simulink model "v00_0A_0D"  (R2022b)
settings: Solver=FixedStepDiscrete  StartTime=0.0  StopTime=8000  FixedStep=SampleTime  MaxStep=Contactors_StepTime_msec  RelTol=1e-3  EnableMultiTasking=on
undefined symbols (not defined in the file): A_to_mA, BalancingTempGroup, canChannel, CapacityFactor, CC_Inputs, CellSOC, ChargeState, ContactorsFlags, DiscIntNeverNeededParam, gEN_Contactors_StepTime_msec, Ion, isDynamicCurrentEn, Lithium, maxAllowedImbalance, nCells_parallel, nCells_series, nCellTempGrps, PermanentFailRecoveryTrigger, ProtectionFlags, RBal_ohm, SampleTime, sigbuilder_block, StLineEq_varA, StLineEq_varB, TempSelectForDCL, Thresholds, V_to_mV
libraries: simulink x32, spsIdealSwitchLib x21, spsBatteryLib x20, spsSeriesRLCBranchLib x20, spsVoltageMeasurementLib x20, canmsglib x4, canlib x3, dspstat3 x2, spspowerguiLib x2, spsControlledCurrentSourceLib x1, spsCurrentMeasurementLib x1
(part 7 of 7)

== stateflow chart v00_0A_0D/HighLevelStatemachine/HighLevelStatemachine ==
  state HighLevelStatemachine [parallel]
    settings: executionOrder=1
    state Normal_Mode [group]
      state Idle
        entry: HighLevelState = HighLevelMode.Idle;
      state Discharging
        entry: HighLevelState = HighLevelMode.Discharging;
      state FastCharging
        entry: HighLevelState = HighLevelMode.ChargingFast;
      state SlowCharging
        entry: HighLevelState = HighLevelMode.ChargingSlow;
      state Regeneration
        entry: HighLevelState = HighLevelMode.Regeneration;
      (default) -> HighLevelStatemachine.Normal_Mode.Idle
      HighLevelStatemachine.Normal_Mode.Idle -> Discharging [order 1] : [duration(DataPipeline.isChargeEn ==0, msec)>Thresholds.NormalModeTimeout_msec]
      Discharging -> HighLevelStatemachine.Normal_Mode.Idle [order 2] : [duration(DataPipeline.Current_mA < Thresholds.ChargeDetectionThreshold_mA, msec) > Thresholds.NormalModeTimeout_msec]
      FastCharging -> Discharging [order 3] : [duration(DataPipeline.isChargeEn ==0, msec)>Thresholds.NormalModeTimeout_msec]
      FastCharging -> HighLevelStatemachine.Normal_Mode.Idle [order 2] : [duration(DataPipeline.Current_mA < Thresholds.ChargeDetectionThreshold_mA, msec) > Thresholds.NormalModeTimeout_msec]
      Discharging -> SlowCharging [order 1] : [duration(DataPipeline.isChargeEn ==1, msec)>Thresholds.NormalModeTimeout_msec]
      SlowCharging -> Discharging [order 4] : [duration(DataPipeline.isChargeEn ==0, msec)>Thresholds.NormalModeTimeout_msec]
      Discharging -> Regeneration [order 3] : [duration((DataPipeline.VCU.isChargerConnected == 0 && DataPipeline.isChargeEn ==1), msec)>Thresholds.NormalModeTimeout_msec]
      Regeneration -> Discharging [order 1] : [duration(DataPipeline.isChargeEn == 0, msec)> Thresholds.NormalModeTimeout_msec]
      HighLevelStatemachine.Normal_Mode.Idle -> SlowCharging [order 2] : [duration(DataPipeline.isChargeEn ==1, msec)>Thresholds.NormalModeTimeout_msec]
      SlowCharging -> HighLevelStatemachine.Normal_Mode.Idle [order 2] : [duration(DataPipeline.Current_mA < Thresholds.ChargeDetectionThreshold_mA, msec) > Thresholds.NormalModeTimeout_msec]
      SlowCharging -> FastCharging [order 1] : [duration(DataPipeline.VCU.FastCharge == 1, msec)>Thresholds.NormalModeTimeout_msec ]
      FastCharging -> SlowCharging [order 1] : [duration(DataPipeline.VCU.SlowCharge == 1, msec)>Thresholds.NormalModeTimeout_msec ]
    state PowerSaver_Mode [group]
      state LowPowerMode
        entry: HighLevelState = HighLevelMode.LowPowerMode;
      state DeepSleepMode
        entry: HighLevelState = HighLevelMode.DeepSleepMode;
      LowPowerMode -> DeepSleepMode : [duration(HighLevelState == HighLevelMode.LowPowerMode, msec) > Thresholds.PowerSaverModeTimeout_msec]
    state Fault_Mode
      state PermanentFailure
        HighLevelState = HighLevelMode.PermanentFailFault;
      state Protection
        HighLevelState = HighLevelMode.ProtectionFault;
      state LimpHome
        HighLevelState = HighLevelMode.LimpHomeFault;
      LimpHome -> PermanentFailure [order 1] : [duration(DataPipeline.VCU.VCUPermanentFail ==1, msec)> Thresholds.FaultsModeTimeout_msec]
      Protection -> LimpHome [order 1] : [duration(DataPipeline.VCU.TransmissionFail ==1 , msec)> Thresholds.FaultsModeTimeout_msec]
    state Service_Mode [group]
      state ServiceMode
        entry: HighLevelState = HighLevelMode.ServiceMode;
    HighLevelStatemachine.Normal_Mode.Idle -> ServiceMode [order 4] : [duration(DataPipeline.VCU.ServiceMode==1,msec)>Thresholds.ServiceModeTimeout_msec]
    Discharging -> Protection [order 4] : [duration(ProtectionOutput.ErrorDetect ==1,msec)>Thresholds.FaultsModeTimeout_msec]
    HighLevelStatemachine.Normal_Mode.Idle -> LowPowerMode [order 3] : [duration(HighLevelState == HighLevelMode.Idle, msec) > Thresholds.PowerSaverModeTimeout_msec]
    FastCharging -> Protection [order 4] : [duration(ProtectionOutput.ErrorDetect ==1,msec)>Thresholds.FaultsModeTimeout_msec]
    SlowCharging -> Protection [order 3] : [duration(ProtectionOutput.ErrorDetect ==1,msec)>Thresholds.FaultsModeTimeout_msec]
    Regeneration -> Protection [order 2] : [duration(ProtectionOutput.ErrorDetect ==1,msec)>Thresholds.FaultsModeTimeout_msec]
    PermanentFailure -> ServiceMode : [duration(DataPipeline.VCU.ServiceMode==1,msec)>Thresholds.ServiceModeTimeout_msec]
    DeepSleepMode -> ServiceMode : [duration(DataPipeline.VCU.ServiceMode==1,msec)>Thresholds.ServiceModeTimeout_msec]
    Protection -> ServiceMode [order 2] : [duration(DataPipeline.VCU.ServiceMode==1,msec)>Thresholds.ServiceModeTimeout_msec]
    LimpHome -> ServiceMode [order 2] : [duration(DataPipeline.VCU.ServiceMode==1,msec)>Thresholds.ServiceModeTimeout_msec]
  state BMS_State [parallel]
    settings: executionOrder=2
    state Idle
    state Ready
      en:
      BMS_State = BMSState.MARVEL_READY;
    state Activating
      en:
      BMS_State = BMSState.MARVEL_ACTIVATING;
    state Error
      en:
      BMS_State = BMSState.MARVEL_ERROR;
    state Active
      en:
      BMS_State = BMSState.MARVEL_ACTIVE;
    (default) -> BMS_State.Idle
    BMS_State.Idle -> Activating [order 2] : [ContactorCommand==1]
    BMS_State.Idle -> Ready [order 1] : [ContactorCommand==0]
    Ready -> Activating [order 1] : [ContactorsState > 0 && ContactorCommand==1]
    Activating -> Ready [order 3] : [ContactorCommand==0&& ContactorsState==0]
    Activating -> Error [order 2] : [duration(ContactorCommand==1&& (ContactorsState==0 || ContactorsState==8),msec)>Thresholds.BMS_ActivatingToError_Timeout_msec]
    Error -> Ready [order 1] : [ProtectionOutput.ErrorDetect == ProtectionFlags.NoError && ContactorsState == 0 && ContactorCommand==0]
    Ready -> Error [order 2] : [ProtectionOutput.ErrorDetect == ProtectionFlags.Error || ContactorsState >6]
    Active -> Ready [order 2] : [ContactorCommand==0&&ContactorsState~=5]
    Error -> Activating [order 2] : [duration((ContactorCommand==1&&ContactorsState>0&&ContactorsState<=6),msec)>Thresholds.BMS_ErrorToActivating_Timeout_msec]
    Activating -> Active [order 1] : [ContactorsState == 5]
    Active -> Activating [order 3] : [ContactorsState<6 && ContactorCommand==1 && ContactorsState~=5]
    Active -> Error [order 1] : [ContactorCommand==1&&(ContactorsState==0||ContactorsState==8)]
  data: Thresholds input; ContactorCommand input; ContactorsState input; ProtectionOutput input; HighLevelState output Enum: HighLevelMode =HighLevelMode.Idle; DataPipeline input; BMS_State output

== matlab function v00_0A_0D/DataPipeline/AverageFunction ==
  data: u1 input; u2 input; Average output; n input
function Average  = fcn(u1,u2,n)
A = [u1,u2];
Average = mean(A(1:n));
end

== matlab function v00_0A_0D/DataPipeline/MaximumFunction ==
  data: n input; u1 input; u2 input; Max output
function Max  = fcn(n,u1,u2)
A = [u1,u2];
Max = max(A(1:n));
end

== matlab function v00_0A_0D/DataPipeline/DynamicCurrentLimits_perParallelCell ==
  data: DCL_ChargingCurrent_A output; DCL_DisChargingCurrent_A output; DCL_arcReactor_A output; SOC input; Temperature_C input
 function [DCL_ChargingCurrent_A, DCL_DisChargingCurrent_A, DCL_arcReactor_A]= fcn(SOC,Temperature_C)
% DCL_ChargingCurrent_A = (SOC*Temperature_C/20);
% DCL_DisChargingCurrent_A = (SOC*Temperature_C/20);
DCL_ChargingCurrent_A = 120;
DCL_DisChargingCurrent_A = (SOC*Temperature_C/20);
DCL_arcReactor_A = (12);
end

== matlab function v00_0A_0D/DataPipeline/MinimumFunction ==
  data: n input; u1 input; u2 input; Min output
function Min  = fcn(n,u1,u2)
A = [u1,u2];
Min = min(A(1:n));
end

== stateflow chart v00_0A_0D/SOCEstimation/CoulombCounter/Chart1 ==
  state IntegratedCurrent
    during:
    IntegratedCurrent = single(single(LoopTimer_SOC_msec)*single(Current_mA))+IntegratedCurrent;
  state IntegratorReset
    during:
    IntegratedCurrent = 0;
  (default) -> IntegratedCurrent
  IntegratedCurrent -> IntegratorReset : [CC_State ==1]
  IntegratorReset -> IntegratedCurrent : [CC_State ==0 || CC_State ==2]
  data: LoopTimer_SOC_msec input; Current_mA input; IntegratedCurrent output =single(0); CC_State input

== stateflow chart v00_0A_0D/SOCEstimation/SOC_Calibration/SOC_Calibration ==
  state Vehicle_at_Rest
    entry:  CC_State = CCState.Vehicle_at_Rest; % CC_State == 2;
    Initial_Capacity_mAh = int32(Initial_Guess_mAh);
    TransitionCapacity_mAh = Initial_Capacity_mAh;
  state CoulombCounting
    entry:
    CC_State = CCState.CoulombCounting; % CC_State == 0;
    Initial_Capacity_mAh = int32(Capacity_mAh);
    during:
    DeltaCapacity_mAh = int32(abs(Initial_Capacity_mAh - TransitionCapacity_mAh));
  state PseudoLatchHandler
    entry:
    pseudoLatchSuccess = false;
  note: It has to be ensured that at a condition at the following conditions:
      | MaxVoltageLimit_mV
      | MaxCurrentLimit_mA
      | MinCurrentLimit_mA
      | There must be sufficient capacity available in the pack to enable the
      | CapacityDeltaCheck_mAh condition.
  note: [duration(DataPipeline.VoltageSenseBus.mV_min>=(single(CC_Inputs.MaxVoltageLimit_mV) - single(CC_Inputs.MaxAllowedImb_mV)),msec)>CC_Inputs.DebouncingTimeout_msec && DataPipeline.VCU.isChargerConnected == 1 && CellBalancingOutput.MaxImbalance_mV<CC_Inputs.MaxAllowedImb_mV && (duration((abs(Current_mA)<CC_Inputs.MaxCurrentLimit_mA && abs(Current_mA)>CC_Inputs.MinCurrentLimit_mA),msec)>CC_Inputs.DebouncingTimeout_msec)]
  state Recalibrate_Charging
    entry:
    CC_State = CCState.Recalibrate; % CC_State == 1;
    Initial_Capacity_mAh = int32(MaxUsableCapacity_mAh);
    TransitionCapacity_mAh = Initial_Capacity_mAh;
  note: should make pseudoLatchSuccess false after calibration
  (default) -> Vehicle_at_Rest
  CoulombCounting -> PseudoLatchHandler [order 2] : [pseudoLatchSuccess == true]
  Vehicle_at_Rest -> CoulombCounting : [after(CC_Inputs.CCTimeout_msec, msec)]
  Recalibrate_Charging -> CoulombCounting : [after(CC_Inputs.CCTimeout_msec, msec)]
  CoulombCounting -> Recalibrate_Charging [order 1] : [duration(((DataPipeline.VoltageSenseBus.mV_min>=minVoltageForLatch) && (abs(Current_mA)<MaxCurrentLimit_mA && abs(Current_mA)>MinCurrentLimit_mA)),msec)>DebouncingTimeout_msec && DataPipeline.VCU.isChargerConnected == 1 && CellBalancingOutput.MaxImbalance_mV<MaxAllowedImb_mV]
  PseudoLatchHandler -> Recalibrate_Charging
  data: MinCurrentLimit_mA input; MaxUsableCapacity_mAh input; Initial_Guess_mAh input; Current_mA input; CC_Inputs input; DataPipeline input; CellBalancingOutput input; CC_State output Enum: CCState; pseudoLatchSuccess output; Capacity_mAh input; Initial_Capacity_mAh output int32; DeltaCapacity_mAh local; TransitionCapacity_mAh local; minVoltageForLatch input; MaxAllowedImb_mV input; MaxCurrentLimit_mA input; DebouncingTimeout_msec input; pseudoLatchSuccess input

== matlab function v00_0A_0D/DataPipeline/I2t_perParallelCell ==
  data: SOC input; i2t_Charge_A2sec output; Temperature_C input; i2t_Discharge_A2sec output
function [i2t_Charge_A2sec, i2t_Discharge_A2sec]= fcn(SOC,Temperature_C)
    i2t_Charge_A2sec = (SOC*Temperature_C*128);
    i2t_Discharge_A2sec = (SOC*Temperature_C*12);
    % i2t_Charge_mA2msec = SOC*Temperature_C*12;
    % i2t_Discharge_mA2msec = SOC*Temperature_C*12;
end

== matlab function v00_0A_0D/SOCEstimation/SOC_ReadFromFlash ==
  data: CapacityRemains_mAh output
function CapacityRemains_mAh = fcn
w = 165; % random value for trial
CapacityRemains_mAh = int32(w * 1000);
end

== matlab function v00_0A_0D/SOCEstimation/SOC_WriteToFlash ==
  data: A output; SOH_pct input; TotalCapacityExchange_mAh input; MaxUsableCapacity_mAh input; SOC_cpct input; TotalDischarge_mAh input; TotalCapacityRemains_mAh input; XYZ output; SOC output
  function [A,XYZ,SOC] = fcn(SOH_pct,TotalCapacityExchange_mAh, MaxUsableCapacity_mAh,SOC_cpct, TotalDischarge_mAh, TotalCapacityRemains_mAh)
A = single(SOH_pct)*single(TotalDischarge_mAh);
B = single(TotalCapacityExchange_mAh)/single(MaxUsableCapacity_mAh);
C = single(SOC_cpct)-single(TotalCapacityRemains_mAh);
XYZ = A+B+C;
SOC = SOC_cpct;
end

== stateflow chart v00_0A_0D/SOCEstimation/SOH_Calculation/Chart ==
  state IntegratedCurrent
    during:
    IntegratedCurrent = single(single(LoopTimer_SOC_msec)*single(Current_mA))+IntegratedCurrent;
  (default) -> IntegratedCurrent
  data: LoopTimer_SOC_msec input; Current_mA input; IntegratedCurrent output =single(0)

== matlab function v00_0A_0D/SOCEstimation/SOH_Calculation/UsableCapacity_mAh ==
  data: CycleCount input; SOH_Vs_Capacity_Gain input; SOH_Vs_Capacity_Offset input; MaxUsableCapacity_mAh output; InstalledCapacity_mAh input
function MaxUsableCapacity_mAh = fcn(CycleCount, SOH_Vs_Capacity_Gain, SOH_Vs_Capacity_Offset, InstalledCapacity_mAh)
    MaxUsableCapacity_mAh = int32(single(InstalledCapacity_mAh) - (single(SOH_Vs_Capacity_Gain) * (single(CycleCount) + single(SOH_Vs_Capacity_Offset))));
end

== stateflow chart v00_0A_0D/SOCEstimation/SOH_Calibration/SOH_Calibration ==
  state TestBench_Entry
    entry: CycleCompleted = 0;
  state Full_Charge
    entry: CycleCompleted = CycleCompleted + 0.5;
  state Int3
  state Int4
  state Full_Discharge
    entry: CycleCompleted = CycleCompleted + 0.5;
  state Int1
  state Int2
  (default) -> TestBench_Entry
  Int3 -> TestBench_Entry [order 2] : [duration(DataPipeline.isChargeEn == 0,msec)>=CC_Inputs.SOHCalibrationTimeout_msec]{CalcEnable = 0}
  Int3 -> Full_Charge [order 1] : [duration(ProtectionOutput.OV == ProtectionFlags.Error,msec)>=CC_Inputs.SOHCalibrationTimeout_msec]{CalcEnable = 1}
  TestBench_Entry -> Int3 [order 2] : [duration(DataPipeline.isChargeEn == 1,msec)>=CC_Inputs.SOHCalibrationTimeout_msec]{CalcEnable = 1}
  Full_Charge -> TestBench_Entry [order 2] : [duration(DataPipeline.isChargeEn == 0 && ProtectionOutput.OV ~= ProtectionFlags.Error,msec)>=CC_Inputs.SOHCalibrationTimeout_msec]{CalcEnable = 0}
  TestBench_Entry -> Int4 [order 1] : [duration(DataPipeline.isChargeEn == 0,msec)>=CC_Inputs.SOHCalibrationTimeout_msec]{CalcEnable = 1}
  Int4 -> TestBench_Entry [order 2] : [duration(DataPipeline.isChargeEn == 1,msec)>=CC_Inputs.SOHCalibrationTimeout_msec]{CalcEnable = 0}
  Full_Discharge -> TestBench_Entry [order 2] : [duration(DataPipeline.isChargeEn == 1 && ProtectionOutput.UV ~= ProtectionFlags.Error,msec)>=CC_Inputs.SOHCalibrationTimeout_msec]{CalcEnable = 0}
  Int2 -> TestBench_Entry [order 1] : [duration(DataPipeline.isChargeEn == 1,msec)>=CC_Inputs.SOHCalibrationTimeout_msec]{CalcEnable = 0}
  Int1 -> TestBench_Entry [order 2] : [duration(DataPipeline.isChargeEn == 0,msec)>=CC_Inputs.SOHCalibrationTimeout_msec]{CalcEnable = 0}
  Int1 -> Full_Charge [order 1] : [duration(DataPipeline.isChargeEn == 0 && ProtectionOutput.OV == ProtectionFlags.Error, msec) >= CC_Inputs.SOHCalibrationTimeout_msec]{CalcEnable = 1}
  Full_Charge -> Int2 [order 1] : [duration(DataPipeline.isChargeEn == 0,msec)>=CC_Inputs.SOHCalibrationTimeout_msec]{CalcEnable = 1}
  Int4 -> Full_Discharge [order 1] : [duration(ProtectionOutput.UV == ProtectionFlags.Error,msec)>=CC_Inputs.SOHCalibrationTimeout_msec]{CalcEnable = 1}
  Full_Discharge -> Int1 [order 1] : [duration(DataPipeline.isChargeEn == 1,msec)>=CC_Inputs.SOHCalibrationTimeout_msec]{CalcEnable = 1}
  Int2 -> Full_Discharge [order 2] : [duration(DataPipeline.isChargeEn == 0 && ProtectionOutput.UV == ProtectionFlags.Error,msec)>=CC_Inputs.SOHCalibrationTimeout_msec]{CalcEnable = 1}
  data: ProtectionOutput input; CC_Inputs input; DataPipeline input; CalcEnable output; CycleCompleted output

== stateflow chart v00_0A_0D/SOCEstimation/SOH_Calibration/Subsystem/Chart ==
  state IntegratedCurrent
    during:
    IntegratedCurrent = single(single(LoopTimer_SOC_msec)*single(Current_mA))+IntegratedCurrent;
  state Reset_IntegratedCurrent
    entry:
    Final_IntegratedCurrent = IntegratedCurrent;
  (default) -> IntegratedCurrent
  IntegratedCurrent -> Reset_IntegratedCurrent : [duration(CycleCompleted == 1,msec)>=CC_Inputs.SOHCalibrationTimeout_msec]
  Reset_IntegratedCurrent -> IntegratedCurrent : [duration(CycleCompleted == 0, msec)>=CC_Inputs.SOHCalibrationTimeout_msec]{IntegratedCurrent = 0}
  data: LoopTimer_SOC_msec input; Current_mA input; CycleCompleted input; CC_Inputs input; Final_IntegratedCurrent output; IntegratedCurrent local =single(0)

== matlab function v00_0A_0D/SOCEstimation/SOH_Calibration/Subsystem/UsableCapacity_mAh ==
  data: CycleCount input; MaxUsableCapacity_mAh output; InstalledCapacity_mAh input; SOH_Vs_Capacity_Gain input; SOH_Vs_Capacity_Offset input
function MaxUsableCapacity_mAh = fcn(CycleCount, InstalledCapacity_mAh, SOH_Vs_Capacity_Gain, SOH_Vs_Capacity_Offset)
    MaxUsableCapacity_mAh = int32(single(InstalledCapacity_mAh) - (single(SOH_Vs_Capacity_Gain) * (single(CycleCount) + single(SOH_Vs_Capacity_Offset))));
end

== matlab function v00_0A_0D/SOCEstimation/Voltage_Vs_Capacity ==
  data: Voltage_mV input; Capacity_mAh output
function Capacity_mAh = fcn(Voltage_mV)

Capacity_mAh = uint32(Voltage_mV*50);

== stateflow chart v00_0A_0D/SOCEstimation/Chart ==
  state Lobby
    entry: Final_InstalledCapacity_mAh = CC_Inputs.InstalledCapacity_mAh;
  state FirstCycleCompleted
    entry: Final_InstalledCapacity_mAh = Tested_InstalledCapacity_mAh;
  (default) -> Lobby
  Lobby -> FirstCycleCompleted : [duration(CC_Inputs.SOHCalibrationOn == true && CycleCompleted == 1,msec)>CC_Inputs.DebouncingTimeout_msec]
  FirstCycleCompleted -> Lobby : [CC_Inputs.SOHCalibrationOn == false]
  data: CycleCompleted input; Final_InstalledCapacity_mAh output int32; Tested_InstalledCapacity_mAh input; CC_Inputs input

== stateflow chart v00_0A_0D/CellBalancing/InputProcessing/Chart1 ==
  state PCBTemp_Safe
    entry: PCBTemp = true;
  state PCBTemp_Danger
    entry: PCBTemp = false;
  (default) -> PCBTemp_Safe
  PCBTemp_Safe -> PCBTemp_Danger : [DataPipeline.TemperatureSenseBus(2).T_max >= Thresholds.Temperature(2).Protections_OTC_Error_C || DataPipeline.TemperatureSenseBus(2).T_max >= Thresholds.Temperature(2).Protections_OTD_Error_C]
  PCBTemp_Danger -> PCBTemp_Safe : [DataPipeline.TemperatureSenseBus(2).T_max < Thresholds.Temperature(2).Protections_OTC_Error_C || DataPipeline.TemperatureSenseBus(2).T_max < Thresholds.Temperature(2).Protections_OTD_Error_C]
  data: Thresholds input; DataPipeline input; PCBTemp output

== stateflow chart v00_0A_0D/SOCEstimation/CoulombCounter/Chart ==
  state Lobby
    entry:
    during: TotalCapacityRemains_mAh = Initial_Capacity_mAh + IntegratedCurrent;
  state Zero_Charged
    during: TotalCapacityRemains_mAh = 0;
  state PseudoLatchHandler
    during: TotalCapacityRemains_mAh = Initial_Capacity_mAh + IntegratedCurrent;
  state Fully_Charged
    entry: TotalCapacityRemains_mAh = MaxUsableCapacity_mAh;
    during: TotalCapacityRemains_mAh = Initial_Capacity_mAh + IntegratedCurrent;
  (default) -> Lobby
  Lobby -> Zero_Charged [order 2] : [TotalCapacityRemains_mAh <= 0]
  Lobby -> PseudoLatchHandler [order 3] : [duration((pseudoLatchFlag == true && isChargeEn == 1),msec) > debounceTimeout]
  Zero_Charged -> Lobby : [isChargeEn==1]
  PseudoLatchHandler -> Lobby [order 2] : [duration(pseudoLatchFlag == 0,msec) > debounceTimeout]
  Lobby -> Fully_Charged [order 1] : [Initial_Capacity_mAh == MaxUsableCapacity_mAh && CC_State == 1 && pseudoLatchFlag == false]
  Fully_Charged -> Lobby : [CC_State == 0]
  PseudoLatchHandler -> Fully_Charged [order 1] : [duration(TotalCapacityRemains_mAh >= MaxUsableCapacity_mAh,msec) > debounceTimeout]{pseudoLatchSuccess = true}
  data: isChargeEn input; Initial_Capacity_mAh input; CC_State input; debounceTimeout input; IntegratedCurrent input; TotalCapacityRemains_mAh output =int32(2); MaxUsableCapacity_mAh input; pseudoLatchFlag input; pseudoLatchSuccess output

== stateflow chart v00_0A_0D/HearbeatMonitoring_Configuration/Chart ==
  state Hardware_NoError
    entry: HardwareError = ProtectionFlags.NoError;
  state Hardware_YesError
    entry: HardwareError = ProtectionFlags.Error;
  (default) -> Hardware_NoError
  Hardware_NoError -> Hardware_YesError : [duration(Status==0,msec)>=Thresholds.HardwareError_Timeout_msec]
  data: Status input; Thresholds input; HardwareError output

== stateflow chart v00_0A_0D/HeartbeatMonitoring_Initial/Chart ==
  state HeartbeatCheck_Normal
    entry:
    CAN_Transmission = ProtectionFlags.NoError;
  state HeartbeatCheck_Fail
    entry:
    CAN_Transmission = ProtectionFlags.PermanentFail;
  (default) -> HeartbeatCheck_Normal
  HeartbeatCheck_Normal -> HeartbeatCheck_Fail : [ClockTime > (HeartbeatCounter + 5)]
  data: HeartbeatCounter input; ClockTime input; CAN_Transmission output =ProtectionFlags.NoError

== stateflow chart v00_0A_0D/Protection/Chart ==
  state Integrator_On
    entry:
    m = 1;
    Trigger = 0;
  state Integrator_Reset
    entry:
    m = 0;
    Trigger = 1;
  (default) -> Integrator_On
  Integrator_On -> Integrator_Reset : [duration(m == 1,msec) == AverageTime_msec]
  Integrator_Reset -> Integrator_On : after(10,msec)
  data: Trigger output; m local =uint8(0); AverageTime_msec input

== stateflow chart v00_0A_0D/ChargingAlgorithm/IRCalc ==
  state IRLobby
    en:
    firstVolt = int32(0);
    secondVolt = int32(0);
    thirdVolt = int32(0);
    firstRequestedCurrent = int32(10);
    secondRequestedCurrent= int32(0);
    thirdRequestedCurrent= int32(0);
    internalResistancePulseCurrent = ChargingRequestedCurrent;
  state IRCalculation
    state ResetIRCycleCount
      du:
      if IRComplete == true
      EraseRecordedCycleCount = 1;
      end
    state IRCalcBegin
      du:
      firstRequestedCurrent = DataPipeline.Current_mA;
      firstVolt = DataPipeline.TerminalVoltage_mV;
      internalResistancePulseCurrent = ChargingRequestedCurrent;
    state UpSense
      du:
      thirdVolt = DataPipeline.TerminalVoltage_mV;
      thirdRequestedCurrent = DataPipeline.Current_mA;
    state DropPulse
      du:
      internalResistancePulseCurrent = 0;
    state DropSense
      du:
      secondVolt = DataPipeline.TerminalVoltage_mV;
      secondRequestedCurrent = DataPipeline.Current_mA;
      internalResistancePulseCurrent = ChargingRequestedCurrent;
    (default) -> IRCalcBegin
    UpSense -> ResetIRCycleCount : [after(Thresholds.IRTransition_msec,msec)]
    IRCalcBegin -> DropPulse : [after(Thresholds.IRTransition_msec,msec)]
    DropSense -> UpSense : [after(Thresholds.IRTransition_msec,msec)]
    DropPulse -> DropSense : [after(Thresholds.IRPulseDropTime_sec,sec)]
  state Entry
  (default) -> IRLobby
  IRLobby -> Entry
  Entry -> IRCalculation : [duration((DataPipeline.VCU.isChargerConnected==true &&...
      | (DataPipeline.VCU.SlowCharge==true ||....
      |  DataPipeline.VCU.FastCharge==true) && IRComplete == false),msec) >= Thresholds.IRTransition_msec]
  IRCalculation -> Entry : [duration((DataPipeline.VCU.isChargerConnected==false ||...
      | (DataPipeline.VCU.SlowCharge==false ||....
      |  DataPipeline.VCU.FastCharge==false)&& IRComplete == false),msec) >= Thresholds.IRTransition_msec]
  data: DataPipeline input; IRComplete input; Thresholds input; internalResistancePulseCurrent output; secondRequestedCurrent output; firstRequestedCurrent output; secondVolt output; firstVolt output; thirdVolt output; thirdRequestedCurrent output; ChargingRequestedCurrent input; EraseRecordedCycleCount output

== stateflow chart v00_0A_0D/ChargingAlgorithm/ChargingAlgorithmstep2 ==
  state chargingLobby
    en:
    Constant_K = double(0);
    trickleChargingEnabled = false;
  state TrickleCharging
    state TrickleChargeDisabled
      en:
      du:
      trickleChargingEnabled = false;
    state TrickleChargeEnabled
      en:
      du:
      trickleChargingEnabled = true;
    (default) -> TrickleChargeDisabled
    TrickleChargeDisabled -> TrickleChargeEnabled [order 1] : [DataPipeline.VoltageSenseBus.mV_min <= Thresholds.trickleChargingLimit]
    TrickleChargeEnabled -> TrickleChargeDisabled : [[DataPipeline.VoltageSenseBus.mV_min > Thresholds.trickleChargingLimit]]
  state NormalCharging
    du:
    state FastCharging
      en:
      du:
      state CC
        en:
        du:
        Constant_K = Thresholds.FastCharge_CC_K;
      state CV
        en:
        du:
        Constant_K = Thresholds.FastCharge_CV_K;
        cvModeActivated = true;
      (default) -> NormalCharging.FastCharging.CC
      NormalCharging.FastCharging.CC -> NormalCharging.FastCharging.CV : [DataPipeline.VoltageSenseBus.mV_max >= Thresholds.transitionVoltageCV]
    state SlowCharging
      en:
      du:
      state CC
        en:
        du:
        Constant_K = Thresholds.SlowCharge_CC_K;
      note: CV mode latch condition handled here by default
      state CV
        en:
        du:
        Constant_K = Thresholds.SlowCharge_CV_K;
        cvModeActivated = true;
      (default) -> NormalCharging.SlowCharging.CC
      NormalCharging.SlowCharging.CC -> NormalCharging.SlowCharging.CV : [DataPipeline.VoltageSenseBus.mV_max >= Thresholds.transitionVoltageCV]
    FastCharging -> SlowCharging : [duration((DataPipeline.VCU.SlowCharge == true && DataPipeline.VCU.FastCharge == true),msec)>=Thresholds.ChargeAlgorithm.TransitionTimeout_msec]
    SlowCharging -> FastCharging : [duration((DataPipeline.VCU.FastCharge == true && DataPipeline.VCU.SlowCharge == false),msec)>=Thresholds.ChargeAlgorithm.TransitionTimeout_msec]
  (default) -> chargingLobby
  chargingLobby -> TrickleCharging : [duration(ChargingState ~= ChargeState.NoCharging, msec) >= Thresholds.ChargeAlgorithm.TransitionTimeout_msec]
  TrickleChargeDisabled -> SlowCharging [order 3] : [duration(ChargingState == ChargeState.SlowCharging && ~trickleChargingEnabled,msec)>= Thresholds.ChargeAlgorithm.TransitionTimeout_msec]
  TrickleChargeDisabled -> FastCharging [order 2] : [duration(ChargingState == ChargeState.FastCharging && ~trickleChargingEnabled,msec)>= Thresholds.ChargeAlgorithm.TransitionTimeout_msec]
  TrickleCharging -> chargingLobby : [duration(ChargingState == ChargeState.NoCharging, msec) >= Thresholds.ChargeAlgorithm.TransitionTimeout_msec]{Constant_K = double(0)}
  NormalCharging -> TrickleCharging [order 2] : [duration(DataPipeline.VoltageSenseBus.mV_min < Thresholds.trickleChargingLimit, msec) >= Thresholds.ChargeAlgorithm.TransitionTimeout_msec]
  NormalCharging -> chargingLobby [order 1] : [duration(ChargingState == ChargeState.NoCharging, msec) >= Thresholds.ChargeAlgorithm.TransitionTimeout_msec]{Constant_K = double(0)}
  data: ChargingState input; DataPipeline input; Thresholds input; Constant_K output; maxAllowedImb_mv input; cvModeActivated output; trickleChargingEnabled output =false

== stateflow chart v00_0A_0D/ChargingAlgorithm/ChargingAlgorithmstep1 ==
  state NoCharge
    en:
    IRSlowGuard = false;
    IRFastGuard = false;
    ChargingState = ChargeState.NoCharging;
    IRComplete = false;
  note: ADD
      | if soc mod set chargestatemode
      | else do nothing
      |
      | handle back from ir reset the chargestatemode
  state FastCharge
    en:
    %ChargeStateMode = 0;
    ChargingState = ChargeState.FastCharging;
    du:
    %ChargeStateMode = 2;
    if CC_Outputs.SOC_cpct <= 45
    IRFastGuard = true;
    IRComplete = false;
    end
  state SlowCharge
    en:
    %ChargeStateMode = 0;
    ChargingState = ChargeState.SlowCharging;
    du:
    %ChargeStateMode = 2;
    if CC_Outputs.SOC_cpct <= 45
    IRSlowGuard = true;
    IRComplete = false;
    end
  note: During conditions to be added ?
      | Function for IRGuards
      | Verify and change Scope of IRGuards in symbols plane
      | Temperaturre Dependance needed?
  state IRCalc [commented out]
    en:
    ChargingState = ChargeState.IR_Measurement;
  IRCalc -> NoCharge [commented out] : [DataPipeline.VCU.isChargerConnected==false||(DataPipeline.VCU.SlowCharge==false || DataPipeline.VCU.FastCharge==false)]...
      | {IRFastGuard = false;IRSlowGuard = false;}
  (default) -> NoCharge
  FastCharge -> NoCharge [order 1] : [DataPipeline.VCU.isChargerConnected==false||(DataPipeline.VCU.SlowCharge==false && DataPipeline.VCU.FastCharge==false)]
  SlowCharge -> NoCharge [order 1] : [DataPipeline.VCU.isChargerConnected==false||(DataPipeline.VCU.SlowCharge==false && DataPipeline.VCU.FastCharge==false)]
  NoCharge -> SlowCharge [order 1] : [DataPipeline.VCU.isChargerConnected == true && DataPipeline.VCU.SlowCharge ==true]
  NoCharge -> FastCharge [order 2] : [DataPipeline.VCU.isChargerConnected == true && DataPipeline.VCU.FastCharge ==true]
  FastCharge -> SlowCharge [order 2] : [DataPipeline.VCU.SlowCharge==true && DataPipeline.VCU.FastCharge==false]
  SlowCharge -> FastCharge [order 2] : [DataPipeline.VCU.FastCharge == true && DataPipeline.VCU.SlowCharge ==false]
  IRCalc -> SlowCharge [commented out] : [IRComplete == true && IRSlowGuard == true]{IRSlowGuard = false;}
  SlowCharge -> IRCalc [commented out] : [(((mod(CC_Outputs.SOC_cpct, 50) == 0) && DataPipeline.RecordedCycleCount >= Thresholds.IRCycleCount && IRSlowGuard == true && IRComplete == false) == true) && IR_calcEnable]
  FastCharge -> IRCalc [commented out] : [(((mod(CC_Outputs.SOC_cpct, 50) == 0) && DataPipeline.RecordedCycleCount >= Thresholds.IRCycleCount && IRFastGuard == true && IRComplete == false) == true) && IR_calcEnable]
  IRCalc -> FastCharge [commented out] : [IRComplete == true && IRFastGuard == true]{IRFastGuard = false;}
  data: CC_Outputs input; Thresholds input; DataPipeline input; ChargingState output; IRComplete output; IRFastGuard local boolean; IRSlowGuard local boolean; IR_calcEnable input
